simulink model "phan1_bai2a_kieu1"  (R2019a)
settings: Solver=VariableStepAuto  StartTime=0.0  StopTime=30  RelTol=1e-3
values from neighbouring files (symbols this model uses):
  Tstep = 0.01    [phan1_bai2a_kieu1_test.m]    (also in phan1_bai2a_kieu2_test.m; phan1_bai2b_kieu1_test.m; phan1_bai2b_kieu2_test.m; phan1_bai2c_kieu1_test.m)
libraries: simulink x1
settings Model: Creator=inhuo  LastModifiedBy=inhuo

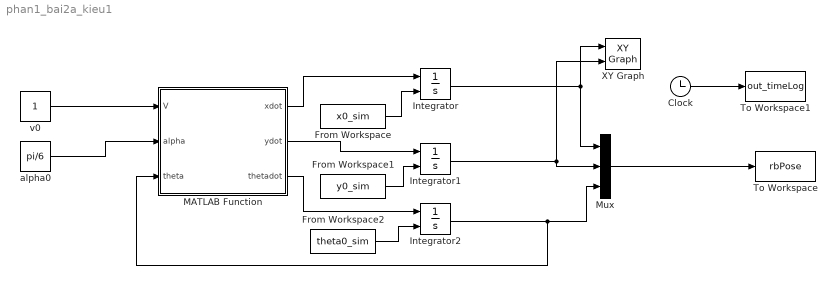
== system phan1_bai2a_kieu1 ==
  Clock : Clock
  From Workspace : FromWorkspace  VariableName=x0_sim  SampleTime=0  OutputAfterFinalValue=Holding final value
  From Workspace1 : FromWorkspace  VariableName=y0_sim  SampleTime=0  OutputAfterFinalValue=Holding final value
  From Workspace2 : FromWorkspace  VariableName=theta0_sim  SampleTime=0  OutputAfterFinalValue=Holding final value
  Integrator : Integrator  InitialConditionSource=external
  Integrator1 : Integrator  InitialConditionSource=external
  Integrator2 : Integrator  InitialConditionSource=external
  MATLAB Function : MATLAB Function  TreatAsAtomicUnit=on
  Mux : Mux  Inputs=3
  To Workspace : ToWorkspace  VariableName=rbPose  SampleTime=Tstep
  To Workspace1 : ToWorkspace  VariableName=out_timeLog  SampleTime=-1
      settings: Save2DSignal=2-D array (concatenate along first dimension)
  XY Graph : simulink/Sinks/XY Graph  xmin=-5  xmax=5  ymin=0  ymax=10  st=-1
  alpha0 : Constant  Value=pi/6
  v0 : Constant
  wires:
  Integrator2/1 -> MATLAB Function/3(theta), Mux/3
  v0/1 -> MATLAB Function/1(V)
  MATLAB Function/2(ydot) -> Integrator1/1
  Integrator/1 -> Mux/1, XY Graph/1
  MATLAB Function/3(thetadot) -> Integrator2/1
  Integrator1/1 -> Mux/2, XY Graph/2
  alpha0/1 -> MATLAB Function/2(alpha)
  MATLAB Function/1(xdot) -> Integrator/1
  Mux/1 -> To Workspace/1
  Clock/1 -> To Workspace1/1
  From Workspace/1 -> Integrator/2
  From Workspace1/1 -> Integrator1/2
  From Workspace2/1 -> Integrator2/2

== matlab function phan1_bai2a_kieu1/MATLAB Function ==
  data: V input; xdot output; alpha input; theta input; ydot output; thetadot output
function [xdot , ydot , thetadot]= fcn(V,alpha,theta)

    d = sqrt (2.5 + 0.1*9);

    if abs(alpha)>pi/4
        alpha = pi/4*sign(alpha);
    end

    if V > (1.5 + 0.03 * 9) %lon hon van toc cuc dai
        V = (1.5 + 0.03 * 9)
    end

     %case 1 : kieu 1
     xdot = V*cos(alpha)*cos(theta);
     ydot = V*cos(alpha)*sin(theta);
     thetadot =V*sin(alpha)/d;
     
end


% case 1 
% xdot = V*cos(alpha)*cos(theta);
% ydot = V*cos(alpha)*sin(theta);
% thetadot =V*sin(alpha)/d;

% case 2
% xdot = V*cos(theta);
% ydot = V*sin(theta);
% thetadot =V*tan(alpha)/d;
